simulink model "PTMotorCU"  (Simulink 7.5)
settings: Solver=ode45  StartTime=0.0  StopTime=inf  RelTol=1e-3
PreLoadFcn:
  | xData = [0 13.5 21 35 50 100];
  | yData = [150 150 95 57 39 20];
InitFcn:
  | xData = [0 0.128];
  | yData = [150 150];
libraries: simulink x7, CarMaker4SL x1
(part 1 of 2)
settings Model: Creator=fh  LastModifiedBy=ml  ExtModeAutoUpdateStatusClock=off
settings DataIOCC: SignalLoggingName=sigsOut
settings OptimizationCC: BooleanDataType=off  InitFltsAndDblsToZero=on
settings DebuggingCC: SaveWithParameterizedLinksMsg=none  SignalResolutionControl=TryResolveAllWithWarning  SolverPrmCheckMsg=none  MultiTaskDSMMsg=warning  MultiTaskCondExecSysMsg=none
settings HardwareCC: TargetUnknown=on
settings RTWCC: IncludeERTFirstTime=on
settings CodeAppCC: MaxIdLength=63
settings GRTTargetCC: TargetFcnLib=ansi_tfl_tmw.mat

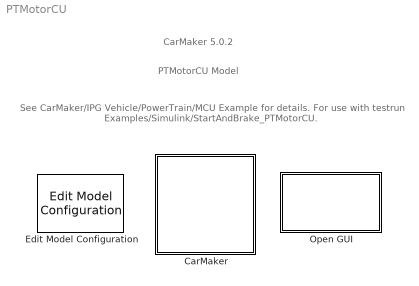
== system PTMotorCU ==
  note: PTMotorCU Model
  note: See CarMaker/IPG Vehicle/PowerTrain/MCU Example for details.
      | For use with testrun Examples/Simulink/StartAndBrake_PTMotorCU.
  note: CarMaker 5.0.2
  CarMaker : Subsystem  TreatAsAtomicUnit=on
      mask Display: image(imread('CarMaker4SLss.bmp'));
  Edit Model Configuration : CarMaker4SL/Edit Model Configuration
  Open GUI : Subsystem  LoadFcn=if ~length(which('cmcmd')), cmenv; end
      settings: OpenFcn=cmblockmagic('gui_fix_display'); CM_Simulink
      mask Display: image(imread('CarMakerGUI.bmp'));

== system PTMotorCU/CarMaker ==
  CM_FIRST : Subsystem
  CM_LAST : Subsystem
  DrivMan : Subsystem
  Ground : Ground
  IPG Vehicle : Subsystem  TreatAsAtomicUnit=on
  Terminator : Terminator
  VehicleControl : Subsystem
  wires:
  DrivMan/2(DrivMan.Out) -> VehicleControl/2(DrivMan.In)
  DrivMan/1(Sync_Out) -> VehicleControl/1(Sync_In)
  CM_FIRST/2(Env.Misc) -> DrivMan/2(Env.Misc)
  CM_FIRST/1(Sync_Out) -> DrivMan/1(Sync_In)
  CM_LAST/1(Sync_Out) -> Terminator/1
  Ground/1 -> CM_FIRST/1(Sync_In)
  IPG Vehicle/1(Sync_Out) -> CM_LAST/1(Sync_In)
  VehicleControl/1(Sync_Out) -> IPG Vehicle/1(Sync_In)
  VehicleControl/3(VhclCtrl.Steering) -> IPG Vehicle/3(VhclCtrl.Steering)
  VehicleControl/4(Vhcl.Wheel.In) -> IPG Vehicle/4(Vhcl.Wheel.In)
  VehicleControl/5(Vhcl.Misc) -> IPG Vehicle/5(Vhcl.Misc)
  VehicleControl/6(VhclCtrl.Brake) -> IPG Vehicle/6(VhclCtrl.Brake)
  VehicleControl/7(VhclCtrl.PT) -> IPG Vehicle/7(VhclCtrl.PT)
  VehicleControl/2(Vhcl.Model.Source) -> IPG Vehicle/2(Vhcl.Model.Source)

== system PTMotorCU/Open GUI ==
  S-Function : S-Function  FunctionName=cm_gui  EnableBusSupport=off

== system PTMotorCU/CarMaker/CM_FIRST ==
  Sync_In : Inport  OutDataType=sfix(16)  OutScaling=2^0
  Bus Creator1 : BusCreator  Inputs=9
  Demux : Demux  Outputs=9
  Environment : S-Function  FunctionName=CM_Sfun  Parameters='Environment'  EnableBusSupport=off
  IoIn : S-Function  FunctionName=CM_Sfun  Parameters='IoIn'  EnableBusSupport=off
  Sync_Out : Outport  OutDataType=sfix(16)  OutScaling=2^0
  Env.Misc : Outport  Port=2  OutDataType=sfix(16)  OutScaling=2^0
  wires:
  Demux/9 -> Bus Creator1/9  "Env WindVel_tot z"
  Demux/8 -> Bus Creator1/8  "Env WindVel_tot y"
  Demux/7 -> Bus Creator1/7  "Env WindVel_tot x"
  Demux/6 -> Bus Creator1/6  "Env SolarRadiation"
  Demux/5 -> Bus Creator1/5  "Env Time"
  Sync_In/1 -> IoIn/1
  IoIn/1 -> Environment/1
  Environment/1 -> Sync_Out/1
  Demux/1 -> Bus Creator1/1  "Env Temperature"
  Demux/2 -> Bus Creator1/2  "Env AirDensity"
  Demux/3 -> Bus Creator1/3  "Env AirPressure"
  Demux/4 -> Bus Creator1/4  "Env AirHumidity"
  Environment/2 -> Demux/1
  Bus Creator1/1 -> Env.Misc/1

== system PTMotorCU/CarMaker/CM_LAST ==
  Sync_In : Inport  OutDataType=sfix(16)  OutScaling=2^0
  CM_User : S-Function  FunctionName=CM_Sfun  Parameters='CM_User'  EnableBusSupport=off
  IoOut : S-Function  FunctionName=CM_Sfun  Parameters='IoOut'  EnableBusSupport=off
  Sync_Out : Outport  OutDataType=sfix(16)  OutScaling=2^0
  wires:
  IoOut/1 -> Sync_Out/1
  CM_User/1 -> IoOut/1
  Sync_In/1 -> CM_User/1

== system PTMotorCU/CarMaker/DrivMan ==
  note: There's rarely a reason to override DrivMan signals.
      | Use the VehicleControl interface for this purpose.
  Sync_In : Inport  OutDataType=sfix(16)  OutScaling=2^0
  Env.Misc : Inport  Port=2  OutDataType=sfix(16)  OutScaling=2^0
  BusCreator : BusCreator  Inputs=17
  Demux : Demux  Outputs=17
  DrivMan : S-Function  FunctionName=CM_Sfun  Parameters='DrivMan'  EnableBusSupport=off
  Sync_Out : Outport  OutDataType=sfix(16)  OutScaling=2^0
  DrivMan.Out : Outport  Port=2  OutDataType=sfix(16)  OutScaling=2^0
  wires:
  DrivMan/2 -> Demux/1
  BusCreator/1 -> DrivMan.Out/1
  DrivMan/1 -> Sync_Out/1
  Sync_In/1 -> DrivMan/1
  Env.Misc/1 -> DrivMan/2
  Demux/1 -> BusCreator/1  "DrivMan SST"
  Demux/2 -> BusCreator/2  "DrivMan Key"
  Demux/3 -> BusCreator/3  "DrivMan UserSignal0"
  Demux/4 -> BusCreator/4  "DrivMan UserSignal1"
  Demux/5 -> BusCreator/5  "DrivMan UserSignal2"
  Demux/6 -> BusCreator/6  "DrivMan UserSignal3"
  Demux/7 -> BusCreator/7  "DrivMan UserSignal4"
  Demux/8 -> BusCreator/8  "DrivMan SelectorCtrl"
  Demux/9 -> BusCreator/9  "DrivMan GearNo"
  Demux/10 -> BusCreator/10  "DrivMan Brake"
  Demux/11 -> BusCreator/11  "DrivMan BrakePark"
  Demux/12 -> BusCreator/12  "DrivMan Clutch"
  Demux/13 -> BusCreator/13  "DrivMan Gas"
  Demux/14 -> BusCreator/14  "DrivMan Steering Ang"
  Demux/15 -> BusCreator/15  "DrivMan Steering AngVel"
  Demux/16 -> BusCreator/16  "DrivMan Steering AngAcc"
  Demux/17 -> BusCreator/17  "DrivMan Steering Trq"

== system PTMotorCU/CarMaker/IPG Vehicle ==
  Sync_In : Inport  OutDataType=sfix(16)  OutScaling=2^0
  Vhcl.Model.Source : Inport  Port=2  OutDataType=sfix(16)  OutScaling=2^0
  VhclCtrl.Steering : Inport  Port=3  OutDataType=sfix(16)  OutScaling=2^0
  Vhcl.Wheel.In : Inport  Port=4  OutDataType=sfix(16)  OutScaling=2^0
  Vhcl.Misc : Inport  Port=5  OutDataType=sfix(16)  OutScaling=2^0
  VhclCtrl.Brake : Inport  Port=6  OutDataType=sfix(16)  OutScaling=2^0
  VhclCtrl.PT : Inport  Port=7  OutDataType=sfix(16)  OutScaling=2^0
  Brake : Subsystem
  CarAndTrailer : Subsystem
  PowerTrain : Subsystem
  Stop Simulation : Stop
  VehicleSource_BuiltIn : simulink/Logic and Bit Operations/Compare To Constant  SystemSampleTime=-1  relop=~=  const=1  LogicOutDataTypeMode=boolean  ZeroCross=off
  Sync_Out : Outport  OutDataType=sfix(16)  OutScaling=2^0
  wires:
  VhclCtrl.PT/1 -> PowerTrain/3(VhclCtrl.PT)
  CarAndTrailer/1(Sync_Out) -> Brake/1(Sync_In)
  CarAndTrailer/2(Brake.IF.In) -> Brake/2(Brake.IF.In)
  VhclCtrl.Brake/1 -> Brake/3(VhclCtrl.Brake)
  PowerTrain/1(Sync_Out) -> Sync_Out/1
  Vhcl.Misc/1 -> CarAndTrailer/4(Vhcl.Misc)
  Vhcl.Wheel.In/1 -> CarAndTrailer/3(Vhcl.Wheel.In)
  VhclCtrl.Steering/1 -> CarAndTrailer/2(VhclCtrl.Steering)
  Sync_In/1 -> CarAndTrailer/1(Sync_In)
  Vhcl.Model.Source/1 -> VehicleSource_BuiltIn/1
  VehicleSource_BuiltIn/1 -> Stop Simulation/1
  Brake/1(Sync_Out) -> PowerTrain/1(Sync_In)
  Brake/2(Vhcl.Wheel.PT) -> PowerTrain/2(Vhcl.Wheel.PT)

== system PTMotorCU/CarMaker/VehicleControl ==
  note: <Your model here>
  note: When implementing a vehicle control model,
      | be sure to add '-disablevehiclecontrol' to the command line arguments
      | in the CarMaker Model Configuration block.
      | Otherwise your model will possibly not see the original DrivMan signals
      | on its inputs, but those of a currently activated C-coded vehicle control model instead.
  Sync_In : Inport  OutDataType=sfix(16)  OutScaling=2^0
  DrivMan.In : Inport  Port=2  OutDataType=sfix(16)  OutScaling=2^0
  Bus Creator2 : BusCreator  Inputs=2
  CreateBus Vhcl.Misc : Subsystem
  CreateBus Vhcl.Wheel.In : Subsystem
  CreateBus VhclCtrl : Subsystem
  CreateBus VhclCtrl.PT : Subsystem
  CreateBus VhclCtrl.Steering : Subsystem
  Demux2 : Demux  Outputs=2
  VehicleControl : S-Function  FunctionName=CM_Sfun  Parameters='VehicleControl'  EnableBusSupport=off
  VehicleControlUpd : S-Function  FunctionName=CM_Sfun  Parameters='VehicleControlUpd'  EnableBusSupport=off
  Sync_Out : Outport  OutDataType=sfix(16)  OutScaling=2^0
  Vhcl.Model.Source : Outport  Port=2  OutDataType=sfix(16)  OutScaling=2^0
  VhclCtrl.Steering : Outport  Port=3  OutDataType=sfix(16)  OutScaling=2^0
  Vhcl.Wheel.In : Outport  Port=4  OutDataType=sfix(16)  OutScaling=2^0
  Vhcl.Misc : Outport  Port=5  OutDataType=sfix(16)  OutScaling=2^0
  VhclCtrl.Brake : Outport  Port=6  OutDataType=sfix(16)  OutScaling=2^0
  VhclCtrl.PT : Outport  Port=7  OutDataType=sfix(16)  OutScaling=2^0
  wires:
  CreateBus VhclCtrl/1(Out) -> VehicleControlUpd/2
  VehicleControl/2 -> CreateBus VhclCtrl/1(In)
  VehicleControlUpd/2 -> Vhcl.Model.Source/1
  VehicleControlUpd/4 -> CreateBus Vhcl.Wheel.In/1(In1)
  VehicleControlUpd/5 -> CreateBus Vhcl.Misc/1(In1)
  VehicleControlUpd/6 -> Demux2/1
  VehicleControlUpd/7 -> CreateBus VhclCtrl.PT/1(In1)
  VehicleControlUpd/3 -> CreateBus VhclCtrl.Steering/1(In1)
  CreateBus Vhcl.Misc/1(Out1) -> Vhcl.Misc/1
  CreateBus Vhcl.Wheel.In/1(Out1) -> Vhcl.Wheel.In/1
  DrivMan.In/1 -> VehicleControl/2
  VehicleControl/1 -> VehicleControlUpd/1
  Sync_In/1 -> VehicleControl/1
  CreateBus VhclCtrl.PT/1(Out1) -> VhclCtrl.PT/1
  Bus Creator2/1 -> VhclCtrl.Brake/1
  CreateBus VhclCtrl.Steering/1(Out1) -> VhclCtrl.Steering/1
  VehicleControlUpd/1 -> Sync_Out/1
  Demux2/2 -> Bus Creator2/2  "VhclCtrl BrakePark"
  Demux2/1 -> Bus Creator2/1  "VhclCtrl Brake"

== system PTMotorCU/CarMaker/IPG Vehicle/Brake ==
  note: When replacing the entire braking system,
      | be sure to add '-disablebrake' to the command line arguments
      | in the CarMaker Model Configuration block.
  note: <Your model here>
  Sync_In : Inport  OutDataType=sfix(16)  OutScaling=2^0
  Brake.IF.In : Inport  Port=2  OutDataType=sfix(16)  OutScaling=2^0
  VhclCtrl.Brake : Inport  Port=3  OutDataType=sfix(16)  OutScaling=2^0
  Brake : S-Function  FunctionName=CM_Sfun  Parameters='Brake'  EnableBusSupport=off
  BrakeUpd : S-Function  FunctionName=CM_Sfun  Parameters='BrakeUpd'  EnableBusSupport=off
  BusCreator : BusCreator  Inputs=12
  CreateBus Vhcl.Wheel.PT : Subsystem
  Demux : Demux  Outputs=12
  Sync_Out : Outport  OutDataType=sfix(16)  OutScaling=2^0
  Vhcl.Wheel.PT : Outport  Port=2  OutDataType=sfix(16)  OutScaling=2^0
  wires:
  CreateBus Vhcl.Wheel.PT/1(Out) -> Vhcl.Wheel.PT/1
  BrakeUpd/2 -> CreateBus Vhcl.Wheel.PT/1(In)
  Demux/1 -> BusCreator/1  "Brake IF Trq_WB FL"
  Demux/2 -> BusCreator/2  "Brake IF Trq_WB FR"
  Demux/3 -> BusCreator/3  "Brake IF Trq_WB RL"
  Demux/4 -> BusCreator/4  "Brake IF Trq_WB RR"
  Demux/5 -> BusCreator/5  "Brake IF Trq_PB FL"
  Demux/6 -> BusCreator/6  "Brake IF Trq_PB FR"
  Demux/7 -> BusCreator/7  "Brake IF Trq_PB RL"
  Demux/8 -> BusCreator/8  "Brake IF Trq_PB RR"
  Demux/9 -> BusCreator/9  "Brake IF Trq_Reg_trg FL"
  Demux/10 -> BusCreator/10  "Brake IF Trq_Reg_trg FR"
  Demux/11 -> BusCreator/11  "Brake IF Trq_Reg_trg RL"
  Demux/12 -> BusCreator/12  "Brake IF Trq_Reg_trg RR"
  Sync_In/1 -> Brake/1
  BusCreator/1 -> BrakeUpd/2
  Brake/2 -> Demux/1
  VhclCtrl.Brake/1 -> Brake/3
  Brake.IF.In/1 -> Brake/2
  Brake/1 -> BrakeUpd/1  "Sync"
  BrakeUpd/1 -> Sync_Out/1

== system PTMotorCU/CarMaker/IPG Vehicle/CarAndTrailer ==
  Sync_In : Inport  OutDataType=sfix(16)  OutScaling=2^0
  VhclCtrl.Steering : Inport  Port=2  OutDataType=sfix(16)  OutScaling=2^0
  Vhcl.Wheel.In : Inport  Port=3  OutDataType=sfix(16)  OutScaling=2^0
  Vhcl.Misc : Inport  Port=4  OutDataType=sfix(16)  OutScaling=2^0
  CarAndTrailerUpd : Subsystem
  Forces : Subsystem
  Ground : Ground
  Kinematics : Subsystem
  Kinetics : Subsystem
  Steering : Subsystem
  Terminator : Terminator
  Terminator1 : Terminator
  Trailer : Subsystem
  Sync_Out : Outport  OutDataType=sfix(16)  OutScaling=2^0
  Brake.IF.In : Outport  Port=2  OutDataType=sfix(16)  OutScaling=2^0
  wires:
  Kinematics/9(lBuf) -> Forces/9(lBuf)
  Forces/12(FBuf) -> Kinetics/12(FBuf)
  Kinematics/8(lStabi) -> Forces/8(lStabi)
  Kinematics/1(Sync_Out) -> Forces/1(Sync_In)
  Kinematics/2(TireFL_In) -> Forces/2(TireFL_In)
  Kinematics/3(TireFR_In) -> Forces/3(TireFR_In)
  Kinematics/4(TireRL_In) -> Forces/4(TireRL_In)
  Kinematics/5(TireRR_In) -> Forces/5(TireRR_In)
  Forces/1(Sync_Out) -> Kinetics/1(Sync_In)
  Forces/3(Car.Aero) -> Kinetics/3(Car.Aero)
  Kinematics/7(vDamp) -> Forces/7(vDamp)
  Kinematics/6(lSpring) -> Forces/6(lSpring)
  Forces/2(Car.Virtual) -> Kinetics/2(Car.Virtual)
  Forces/4(Car.Load) -> Kinetics/4(Car.Load)
  Forces/5(TireFL_Out) -> Kinetics/5(TireFL.Out)
  Forces/6(TireFR_Out) -> Kinetics/6(TireFR.Out)
  Forces/7(TireRL_Out) -> Kinetics/7(TireRL.Out)
  Forces/8(TireRR_Out) -> Kinetics/8(TireRR.Out)
  Forces/9(FSpring) -> Kinetics/9(FSpring)
  Forces/10(FDamp) -> Kinetics/10(FDamp)
  Forces/11(FStabi) -> Kinetics/11(FStabi)
  Ground/1 -> CarAndTrailerUpd/10(Vhcl.Fr1A)
  Kinetics/1(Sync_Out) -> Trailer/1(Sync_In)
  Steering/1(Sync_Out) -> Kinematics/1(Sync_In)
  Sync_In/1 -> Steering/1(Sync_In)
  VhclCtrl.Steering/1 -> Steering/2(VhclCtrl.Steering)
  Kinetics/2(Trailer.Load) -> Trailer/2(Trailer.Load)
  Kinetics/3(Car.Hitch) -> Trailer/3(Car.Hitch)
  Kinetics/4(Car.Fr1) -> Trailer/4(Car.Fr1)
  Steering/2(Steer.IF) -> Kinematics/2(Steer.IF)
  Kinetics/5(Car.Trq_T2W) -> Trailer/5(Car.Trq_T2W)
  Kinetics/6(WheelCarrier.Misc) -> Trailer/6(WheelCarrier.Misc)
  Vhcl.Wheel.In/1 -> Terminator/1
  Vhcl.Misc/1 -> Terminator1/1
  CarAndTrailerUpd/1(Sync_Out) -> Sync_Out/1
  CarAndTrailerUpd/2(Brake.IF.In) -> Brake.IF.In/1
  Trailer/1(Sync_Out) -> CarAndTrailerUpd/1(Sync_In)
  Trailer/2(Vhcl.Steering) -> CarAndTrailerUpd/2(Vhcl.Steering)
  Trailer/3(Vhcl.Motion) -> CarAndTrailerUpd/3(Vhcl.Motion)
  Trailer/4(Vhcl.PoI) -> CarAndTrailerUpd/4(Vhcl.PoI)
  Trailer/5(Vhcl.Wheel.FL) -> CarAndTrailerUpd/5(Vhcl.Wheel.FL)
  Trailer/6(Vhcl.Wheel.FR) -> CarAndTrailerUpd/6(Vhcl.Wheel.FR)
  Trailer/7(Vhcl.Wheel.RL) -> CarAndTrailerUpd/7(Vhcl.Wheel.RL)
  Trailer/8(Vhcl.Wheel.RR) -> CarAndTrailerUpd/8(Vhcl.Wheel.RR)
  Trailer/9(Car.Hitch.FrcTrq) -> CarAndTrailerUpd/9(Car.Hitch.FrcTrq)

== system PTMotorCU/CarMaker/IPG Vehicle/PowerTrain ==
  note: <Your model here>
  note: When replacing the entire powertrain,
      | be sure to add '-disablepowertrain' to the command line arguments
      | in the CarMaker Model Configuration block.
  Sync_In : Inport  OutDataType=sfix(16)  OutScaling=2^0
  Vhcl.Wheel.PT : Inport  Port=2  OutDataType=sfix(16)  OutScaling=2^0
  VhclCtrl.PT : Inport  Port=3  OutDataType=sfix(16)  OutScaling=2^0
  BusCreator : BusCreator  Inputs=40
  Demux : Demux  Outputs=40
  MCU Example : Subsystem
  PowerTrain : S-Function  FunctionName=CM_Sfun  Parameters='PowerTrain'  EnableBusSupport=off
  PowerTrainUpd : S-Function  FunctionName=CM_Sfun  Parameters='PowerTrainUpd'  EnableBusSupport=off
  Sync_Out : Outport  OutDataType=sfix(16)  OutScaling=2^0
  wires:
  Vhcl.Wheel.PT/1 -> PowerTrain/2
  VhclCtrl.PT/1 -> PowerTrain/3
  Demux/40 -> BusCreator/40  "PT IF WRR Trq_BrakeReg_max"
  Demux/39 -> BusCreator/39  "PT IF WRR Trq_BrakeReg"
  Demux/38 -> BusCreator/38  "PT IF WRR Trq_Supp2WC"
  Demux/37 -> BusCreator/37  "PT IF WRR Trq_Drive"
  Demux/36 -> BusCreator/36  "PT IF WRR Trq_B2W"
  Demux/35 -> BusCreator/35  "PT IF WRR rotv"
  Demux/34 -> BusCreator/34  "PT IF WRR rot"
  Demux/33 -> BusCreator/33  "PT IF WRL Trq_BrakeReg_max"
  Demux/32 -> BusCreator/32  "PT IF WRL Trq_BrakeReg"
  Demux/31 -> BusCreator/31  "PT IF WRL Trq_Supp2WC"
  Demux/30 -> BusCreator/30  "PT IF WRL Trq_Drive"
  Demux/29 -> BusCreator/29  "PT IF WRL Trq_B2W"
  Demux/28 -> BusCreator/28  "PT IF WRL rotv"
  Demux/27 -> BusCreator/27  "PT IF WRL rot"
  Demux/26 -> BusCreator/26  "PT IF WFR Trq_BrakeReg_max"
  Demux/25 -> BusCreator/25  "PT IF WFR Trq_BrakeReg"
  Demux/24 -> BusCreator/24  "PT IF WFR Trq_Supp2WC"
  Demux/23 -> BusCreator/23  "PT IF WFR Trq_Drive"
  Demux/22 -> BusCreator/22  "PT IF WFR Trq_B2W"
  Demux/21 -> BusCreator/21  "PT IF WFR rotv"
  Demux/20 -> BusCreator/20  "PT IF WFR rot"
  Demux/19 -> BusCreator/19  "PT IF WFL Trq_BrakeReg_max"
  Demux/18 -> BusCreator/18  "PT IF WFL Trq_BrakeReg"
  Demux/17 -> BusCreator/17  "PT IF WFL Trq_Supp2WC"
  Demux/16 -> BusCreator/16  "PT IF WFL Trq_Drive"
  Demux/15 -> BusCreator/15  "PT IF WFL Trq_B2W"
  Demux/14 -> BusCreator/14  "PT IF WFL rotv"
  Demux/13 -> BusCreator/13  "PT IF WFL rot"
  Demux/12 -> BusCreator/12  "PT IF DL_iDiff_mean"
  Demux/11 -> BusCreator/11  "PT IF Trq_Supp2BdyEng y"
  Demux/10 -> BusCreator/10  "PT IF Trq_Supp2BdyEng x"
  Demux/9 -> BusCreator/9  "PT IF Trq_Supp2Bdy1 z"
  Demux/8 -> BusCreator/8  "PT IF Trq_Supp2Bdy1 y"
  Demux/7 -> BusCreator/7  "PT IF Trq_Supp2Bdy1 x"
  Demux/6 -> BusCreator/6  "PT IF Engine_Trq (EngineControl)"
  Demux/5 -> BusCreator/5  "PT IF Engine_rotv"
  Demux/4 -> BusCreator/4  "PT IF GearNo"
  Demux/3 -> BusCreator/3  "PT IF OperationError"
  Demux/2 -> BusCreator/2  "PT IF OperationState"
  Demux/1 -> BusCreator/1  "PT IF Ignition"
  BusCreator/1 -> PowerTrainUpd/2
  PowerTrain/1 -> PowerTrainUpd/1, MCU Example/1(Sync_In)  "Sync"
  PowerTrainUpd/1 -> Sync_Out/1
  PowerTrain/2 -> Demux/1
  Sync_In/1 -> PowerTrain/1

== system PTMotorCU/CarMaker/VehicleControl/CreateBus Vhcl.Misc ==
  In1 : Inport  OutDataType=sfix(16)  OutScaling=2^0
  Bus Creator5 : BusCreator  Inputs=11
  Demux5 : Demux  Outputs=11
  Out1 : Outport  OutDataType=sfix(16)  OutScaling=2^0
  wires:
  Demux5/11 -> Bus Creator5/11  "Vhcl Wind_vel_0 z"
  Demux5/10 -> Bus Creator5/10  "Vhcl Wind_vel_0 y"
  Demux5/9 -> Bus Creator5/9  "Vhcl Wind_vel_0 x"
  Demux5/8 -> Bus Creator5/8  "Vhcl DL2BdyEng y"
  Demux5/7 -> Bus Creator5/7  "Vhcl DL2BdyEng x"
  Demux5/6 -> Bus Creator5/6  "Vhcl TrqDL2Bdy1B z"
  Demux5/5 -> Bus Creator5/5  "Vhcl TrqDL2Bdy1B y"
  Demux5/4 -> Bus Creator5/4  "Vhcl TrqDL2Bdy1B x"
  Demux5/3 -> Bus Creator5/3  "Vhcl Trq_DL2Bdy1 z"
  In1/1 -> Demux5/1
  Bus Creator5/1 -> Out1/1
  Demux5/2 -> Bus Creator5/2  "Vhcl Trq_DL2Bdy1 y"
  Demux5/1 -> Bus Creator5/1  "Vhcl Trq_DL2Bdy1 x"

== system PTMotorCU/CarMaker/VehicleControl/CreateBus Vhcl.Wheel.In ==
  In1 : Inport  OutDataType=sfix(16)  OutScaling=2^0
  Bus Creator1 : BusCreator  Inputs=12
  Demux1 : Demux  Outputs=12
  Out1 : Outport  OutDataType=sfix(16)  OutScaling=2^0
  wires:
  Demux1/12 -> Bus Creator1/12  "Vhcl Wheel RR rotv"
  Demux1/11 -> Bus Creator1/11  "Vhcl Wheel RR Trq_DL2WC"
  Demux1/10 -> Bus Creator1/10  "Vhcl Wheel RR Trq_B2WC"
  Demux1/9 -> Bus Creator1/9  "Vhcl Wheel RL rotv"
  Demux1/8 -> Bus Creator1/8  "Vhcl Wheel RL Trq_DL2WC"
  Demux1/7 -> Bus Creator1/7  "Vhcl Wheel RL Trq_B2WC"
  Demux1/6 -> Bus Creator1/6  "Vhcl Wheel FR rotv"
  Demux1/5 -> Bus Creator1/5  "Vhcl Wheel FR Trq_DL2WC"
  Demux1/4 -> Bus Creator1/4  "Vhcl Wheel FR Trq_B2WC"
  Demux1/3 -> Bus Creator1/3  "Vhcl Wheel FL rotv"
  In1/1 -> Demux1/1
  Bus Creator1/1 -> Out1/1
  Demux1/2 -> Bus Creator1/2  "Vhcl Wheel FL Trq_DL2WC"
  Demux1/1 -> Bus Creator1/1  "Vhcl Wheel FL Trq_B2WC"

== system PTMotorCU/CarMaker/VehicleControl/CreateBus VhclCtrl ==
  In : Inport
  BusCreator : BusCreator  Inputs=29
  Demux : Demux  Outputs=29
  Out : Outport
  wires:
  In/1 -> Demux/1
  BusCreator/1 -> Out/1
  Demux/1 -> BusCreator/1  "VhclCtrl SST"
  Demux/2 -> BusCreator/2  "VhclCtrl Key"
  Demux/3 -> BusCreator/3  "VhclCtrl UserSignal0"
  Demux/4 -> BusCreator/4  "VhclCtrl UserSignal1"
  Demux/5 -> BusCreator/5  "VhclCtrl UserSignal2"
  Demux/6 -> BusCreator/6  "VhclCtrl UserSignal3"
  Demux/7 -> BusCreator/7  "VhclCtrl UserSignal4"
  Demux/8 -> BusCreator/8  "VhclCtrl GearNo"
  Demux/9 -> BusCreator/9  "VhclCtrl SelectorCtrl"
  Demux/10 -> BusCreator/10  "VhclCtrl Brake"
  Demux/11 -> BusCreator/11  "VhclCtrl BrakePark"
  Demux/12 -> BusCreator/12  "VhclCtrl Clutch"
  Demux/13 -> BusCreator/13  "VhclCtrl Gas"
  Demux/14 -> BusCreator/14  "VhclCtrl Steering Ang"
  Demux/15 -> BusCreator/15  "VhclCtrl Steering AngVel"
  Demux/16 -> BusCreator/16  "VhclCtrl Steering AngAcc"
  Demux/17 -> BusCreator/17  "VhclCtrl Steering Trq"
  Demux/18 -> BusCreator/18  "VhclCtrl Lights LowBeam"
  Demux/19 -> BusCreator/19  "VhclCtrl Lights HighBeam"
  Demux/20 -> BusCreator/20  "VhclCtrl Lights Daytime"
  Demux/21 -> BusCreator/21  "VhclCtrl Lights ParkL"
  Demux/22 -> BusCreator/22  "VhclCtrl Lights ParkR"
  Demux/23 -> BusCreator/23  "VhclCtrl Lights IndL"
  Demux/24 -> BusCreator/24  "VhclCtrl Lights IndR"
  Demux/25 -> BusCreator/25  "VhclCtrl Lights FogFrontL"
  Demux/26 -> BusCreator/26  "VhclCtrl Lights FogFrontR"
  Demux/27 -> BusCreator/27  "VhclCtrl Lights FogRear"
  Demux/28 -> BusCreator/28  "VhclCtrl Lights Brake"
  Demux/29 -> BusCreator/29  "VhclCtrl Lights Reverse"

== system PTMotorCU/CarMaker/VehicleControl/CreateBus VhclCtrl.PT ==
  In1 : Inport
  BusCreator : BusCreator  Inputs=11
  Demux : Demux  Outputs=11
  Out1 : Outport
  wires:
  In1/1 -> Demux/1
  BusCreator/1 -> Out1/1
  Demux/1 -> BusCreator/1  "VhclCtrl SST"
  Demux/2 -> BusCreator/2  "VhclCtrl Key"
  Demux/3 -> BusCreator/3  "VhclCtrl UserSignal0"
  Demux/4 -> BusCreator/4  "VhclCtrl UserSignal1"
  Demux/5 -> BusCreator/5  "VhclCtrl UserSignal2"
  Demux/6 -> BusCreator/6  "VhclCtrl UserSignal3"
  Demux/7 -> BusCreator/7  "VhclCtrl UserSignal4"
  Demux/8 -> BusCreator/8  "VhclCtrl GearNo"
  Demux/9 -> BusCreator/9  "VhclCtrl SelectorCtrl"
  Demux/10 -> BusCreator/10  "VhclCtrl Clutch"
  Demux/11 -> BusCreator/11  "VhclCtrl Gas"

== system PTMotorCU/CarMaker/VehicleControl/CreateBus VhclCtrl.Steering ==
  In1 : Inport  OutDataType=sfix(16)  OutScaling=2^0
  Bus Creator : BusCreator  Inputs=5
  Demux : Demux  Outputs=5
  Out1 : Outport  OutDataType=sfix(16)  OutScaling=2^0
  wires:
  In1/1 -> Demux/1
  Bus Creator/1 -> Out1/1
  Demux/1 -> Bus Creator/1  "VhclCtrl Steering Ang"
  Demux/5 -> Bus Creator/5  "VhclCtrl Steering ByTrq"
  Demux/3 -> Bus Creator/3  "VhclCtrl Steering AngAcc"
  Demux/2 -> Bus Creator/2  "VhclCtrl Steering AngVel"
  Demux/4 -> Bus Creator/4  "VhclCtrl Steering Trq"

== system PTMotorCU/CarMaker/IPG Vehicle/Brake/CreateBus Vhcl.Wheel.PT ==
  In : Inport
  BusCreator : BusCreator  Inputs=16
  Demux : Demux  Outputs=16
  Out : Outport
  wires:
  In/1 -> Demux/1
  BusCreator/1 -> Out/1
  Demux/1 -> BusCreator/1  "Vhcl Wheel FL Trq_Brake"
  Demux/2 -> BusCreator/2  "Vhcl Wheel FL Trq_BrakeReg_trg"
  Demux/3 -> BusCreator/3  "Vhcl Wheel FL Trq_T2W"
  Demux/4 -> BusCreator/4  "Vhcl Wheel FL WhlBearing"
  Demux/5 -> BusCreator/5  "Vhcl Wheel FR Trq_Brake"
  Demux/6 -> BusCreator/6  "Vhcl Wheel FR Trq_BrakeReg_trg"
  Demux/7 -> BusCreator/7  "Vhcl Wheel FR Trq_T2W"
  Demux/8 -> BusCreator/8  "Vhcl Wheel FR WhlBearing"
  Demux/9 -> BusCreator/9  "Vhcl Wheel RL Trq_Brake"
  Demux/10 -> BusCreator/10  "Vhcl Wheel RL Trq_BrakeReg_trg"
  Demux/11 -> BusCreator/11  "Vhcl Wheel RL Trq_T2W"
  Demux/12 -> BusCreator/12  "Vhcl Wheel RL WhlBearing"
  Demux/13 -> BusCreator/13  "Vhcl Wheel RR Trq_Brake"
  Demux/14 -> BusCreator/14  "Vhcl Wheel RR Trq_BrakeReg_trg"
  Demux/15 -> BusCreator/15  "Vhcl Wheel RR Trq_T2W"
  Demux/16 -> BusCreator/16  "Vhcl Wheel RR WhlBearing"

== system PTMotorCU/CarMaker/IPG Vehicle/CarAndTrailer/CarAndTrailerUpd ==
  Sync_In : Inport  OutDataType=sfix(16)  OutScaling=2^0
  Vhcl.Steering : Inport  Port=2  OutDataType=sfix(16)  OutScaling=2^0
  Vhcl.Motion : Inport  Port=3  OutDataType=sfix(16)  OutScaling=2^0
  Vhcl.PoI : Inport  Port=4  OutDataType=sfix(16)  OutScaling=2^0
  Vhcl.Wheel.FL : Inport  Port=5  OutDataType=sfix(16)  OutScaling=2^0
  Vhcl.Wheel.FR : Inport  Port=6  OutDataType=sfix(16)  OutScaling=2^0
  Vhcl.Wheel.RL : Inport  Port=7  OutDataType=sfix(16)  OutScaling=2^0
  Vhcl.Wheel.RR : Inport  Port=8  OutDataType=sfix(16)  OutScaling=2^0
  Car.Hitch.FrcTrq : Inport  Port=9  OutDataType=sfix(16)  OutScaling=2^0
  Vhcl.Fr1A : Inport  Port=10  OutDataType=sfix(16)  OutScaling=2^0
  CarAndTrailerUpd : S-Function  FunctionName=CM_Sfun  Parameters='CarAndTrUpd'  EnableBusSupport=off
  CreateBus Brake.IF.In : Subsystem
  Sync_Out : Outport  OutDataType=sfix(16)  OutScaling=2^0
  Brake.IF.In : Outport  Port=2  OutDataType=sfix(16)  OutScaling=2^0
  wires:
  Sync_In/1 -> CarAndTrailerUpd/1
  CarAndTrailerUpd/1 -> Sync_Out/1
  CreateBus Brake.IF.In/1(Out) -> Brake.IF.In/1
  CarAndTrailerUpd/2 -> CreateBus Brake.IF.In/1(In)
  Vhcl.Wheel.RL/1 -> CarAndTrailerUpd/7
  Vhcl.Wheel.RR/1 -> CarAndTrailerUpd/8
  Car.Hitch.FrcTrq/1 -> CarAndTrailerUpd/9
  Vhcl.Wheel.FR/1 -> CarAndTrailerUpd/6
  Vhcl.Wheel.FL/1 -> CarAndTrailerUpd/5
  Vhcl.PoI/1 -> CarAndTrailerUpd/4
  Vhcl.Motion/1 -> CarAndTrailerUpd/3
  Vhcl.Steering/1 -> CarAndTrailerUpd/2
  Vhcl.Fr1A/1 -> CarAndTrailerUpd/10  "user vehicle only"

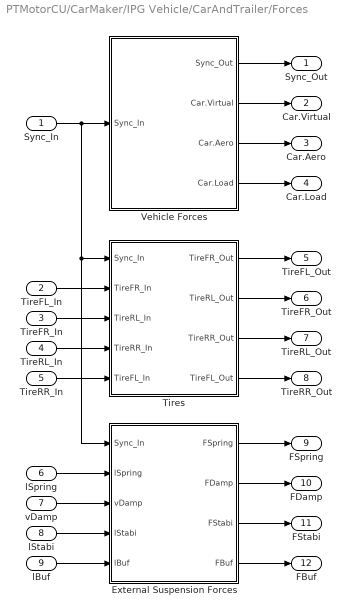
== system PTMotorCU/CarMaker/IPG Vehicle/CarAndTrailer/Forces ==
  Sync_In : Inport  OutDataType=sfix(16)  OutScaling=2^0
  TireFL_In : Inport  Port=2  OutDataType=sfix(16)  OutScaling=2^0
  TireFR_In : Inport  Port=3  OutDataType=sfix(16)  OutScaling=2^0
  TireRL_In : Inport  Port=4  OutDataType=sfix(16)  OutScaling=2^0
  TireRR_In : Inport  Port=5  OutDataType=sfix(16)  OutScaling=2^0
  lSpring : Inport  Port=6  OutDataType=sfix(16)  OutScaling=2^0
  vDamp : Inport  Port=7  OutDataType=sfix(16)  OutScaling=2^0
  lStabi : Inport  Port=8  OutDataType=sfix(16)  OutScaling=2^0
  lBuf : Inport  Port=9  OutDataType=sfix(16)  OutScaling=2^0
  External Suspension Forces : Subsystem
  Tires : Subsystem
  Vehicle Forces : Subsystem
  Sync_Out : Outport  OutDataType=sfix(16)  OutScaling=2^0
  Car.Virtual : Outport  Port=2  OutDataType=sfix(16)  OutScaling=2^0
  Car.Aero : Outport  Port=3  OutDataType=sfix(16)  OutScaling=2^0
  Car.Load : Outport  Port=4  OutDataType=sfix(16)  OutScaling=2^0
  TireFL_Out : Outport  Port=5  OutDataType=sfix(16)  OutScaling=2^0
  TireFR_Out : Outport  Port=6  OutDataType=sfix(16)  OutScaling=2^0
  TireRL_Out : Outport  Port=7  OutDataType=sfix(16)  OutScaling=2^0
  TireRR_Out : Outport  Port=8  OutDataType=sfix(16)  OutScaling=2^0
  FSpring : Outport  Port=9  OutDataType=sfix(16)  OutScaling=2^0
  FDamp : Outport  Port=10  OutDataType=sfix(16)  OutScaling=2^0
  FStabi : Outport  Port=11  OutDataType=sfix(16)  OutScaling=2^0
  FBuf : Outport  Port=12  OutDataType=sfix(16)  OutScaling=2^0
  wires:
  External Suspension Forces/1(FSpring) -> FSpring/1
  External Suspension Forces/3(FStabi) -> FStabi/1
  lStabi/1 -> External Suspension Forces/4(lStabi)
  vDamp/1 -> External Suspension Forces/3(vDamp)
  External Suspension Forces/2(FDamp) -> FDamp/1
  lSpring/1 -> External Suspension Forces/2(lSpring)
  Vehicle Forces/4(Car.Load) -> Car.Load/1
  Vehicle Forces/3(Car.Aero) -> Car.Aero/1
  Vehicle Forces/2(Car.Virtual) -> Car.Virtual/1
  TireFL_In/1 -> Tires/2(TireFR_In)
  Vehicle Forces/1(Sync_Out) -> Sync_Out/1
  Sync_In/1 -> Vehicle Forces/1(Sync_In), Tires/1(Sync_In), External Suspension Forces/1(Sync_In)
  TireFR_In/1 -> Tires/3(TireRL_In)
  TireRL_In/1 -> Tires/4(TireRR_In)
  TireRR_In/1 -> Tires/5(TireFL_In)
  Tires/1(TireFR_Out) -> TireFL_Out/1
  Tires/2(TireRL_Out) -> TireFR_Out/1
  Tires/3(TireRR_Out) -> TireRL_Out/1
  Tires/4(TireFL_Out) -> TireRR_Out/1
  lBuf/1 -> External Suspension Forces/5(lBuf)
  External Suspension Forces/4(FBuf) -> FBuf/1

== system PTMotorCU/CarMaker/IPG Vehicle/CarAndTrailer/Kinematics ==
  Sync_In : Inport  OutDataType=sfix(16)  OutScaling=2^0
  Steer.IF : Inport  Port=2  OutDataType=sfix(16)  OutScaling=2^0
  Kinematics : S-Function  FunctionName=CM_Sfun  Parameters='Kinematics'  EnableBusSupport=off
  Sync_Out : Outport  OutDataType=sfix(16)  OutScaling=2^0
  TireFL_In : Outport  Port=2  OutDataType=sfix(16)  OutScaling=2^0
  TireFR_In : Outport  Port=3  OutDataType=sfix(16)  OutScaling=2^0
  TireRL_In : Outport  Port=4  OutDataType=sfix(16)  OutScaling=2^0
  TireRR_In : Outport  Port=5  OutDataType=sfix(16)  OutScaling=2^0
  lSpring : Outport  Port=6  OutDataType=sfix(16)  OutScaling=2^0
  vDamp : Outport  Port=7  OutDataType=sfix(16)  OutScaling=2^0
  lStabi : Outport  Port=8  OutDataType=sfix(16)  OutScaling=2^0
  lBuf : Outport  Port=9  OutDataType=sfix(16)  OutScaling=2^0
  wires:
  Steer.IF/1 -> Kinematics/2
  Kinematics/1 -> Sync_Out/1
  Sync_In/1 -> Kinematics/1
  Kinematics/7 -> vDamp/1
  Kinematics/6 -> lSpring/1
  Kinematics/5 -> TireRR_In/1
  Kinematics/4 -> TireRL_In/1
  Kinematics/3 -> TireFR_In/1
  Kinematics/2 -> TireFL_In/1
  Kinematics/8 -> lStabi/1
  Kinematics/9 -> lBuf/1

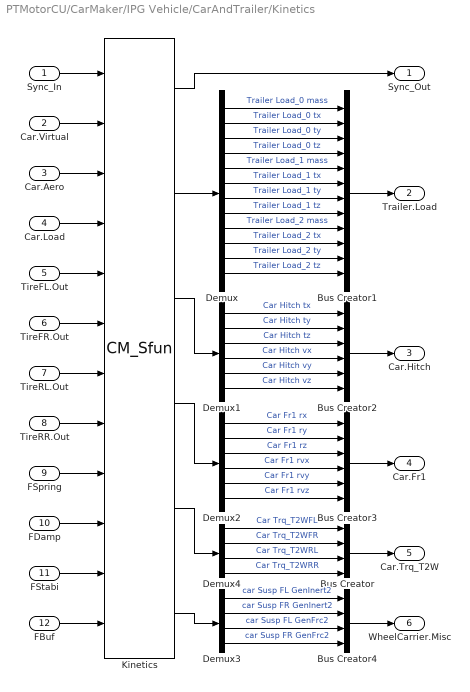
== system PTMotorCU/CarMaker/IPG Vehicle/CarAndTrailer/Kinetics ==
  Sync_In : Inport  OutDataType=sfix(16)  OutScaling=2^0
  Car.Virtual : Inport  Port=2  OutDataType=sfix(16)  OutScaling=2^0
  Car.Aero : Inport  Port=3  OutDataType=sfix(16)  OutScaling=2^0
  Car.Load : Inport  Port=4  OutDataType=sfix(16)  OutScaling=2^0
  TireFL.Out : Inport  Port=5  OutDataType=sfix(16)  OutScaling=2^0
  TireFR.Out : Inport  Port=6  OutDataType=sfix(16)  OutScaling=2^0
  TireRL.Out : Inport  Port=7  OutDataType=sfix(16)  OutScaling=2^0
  TireRR.Out : Inport  Port=8  OutDataType=sfix(16)  OutScaling=2^0
  FSpring : Inport  Port=9  OutDataType=sfix(16)  OutScaling=2^0
  FDamp : Inport  Port=10  OutDataType=sfix(16)  OutScaling=2^0
  FStabi : Inport  Port=11  OutDataType=sfix(16)  OutScaling=2^0
  FBuf : Inport  Port=12  OutDataType=sfix(16)  OutScaling=2^0
  Bus Creator : BusCreator
  Bus Creator1 : BusCreator  Inputs=12
  Bus Creator2 : BusCreator  Inputs=6
  Bus Creator3 : BusCreator  Inputs=6
  Bus Creator4 : BusCreator
  Demux : Demux  Outputs=12
  Demux1 : Demux  Outputs=6
  Demux2 : Demux  Outputs=6
  Demux3 : Demux
  Demux4 : Demux
  Kinetics : S-Function  FunctionName=CM_Sfun  Parameters='Kinetics'  EnableBusSupport=off
  Sync_Out : Outport  OutDataType=sfix(16)  OutScaling=2^0
  Trailer.Load : Outport  Port=2  OutDataType=sfix(16)  OutScaling=2^0
  Car.Hitch : Outport  Port=3  OutDataType=sfix(16)  OutScaling=2^0
  Car.Fr1 : Outport  Port=4  OutDataType=sfix(16)  OutScaling=2^0
  Car.Trq_T2W : Outport  Port=5  OutDataType=sfix(16)  OutScaling=2^0
  WheelCarrier.Misc : Outport  Port=6  OutDataType=sfix(16)  OutScaling=2^0
  wires:
  Kinetics/5 -> Demux4/1
  Kinetics/6 -> Demux3/1
  FStabi/1 -> Kinetics/11
  FDamp/1 -> Kinetics/10
  FSpring/1 -> Kinetics/9
  TireRR.Out/1 -> Kinetics/8
  TireRL.Out/1 -> Kinetics/7
  TireFR.Out/1 -> Kinetics/6
  TireFL.Out/1 -> Kinetics/5
  Demux4/1 -> Bus Creator/1  "Car Trq_T2WFL"
  Demux4/2 -> Bus Creator/2  "Car Trq_T2WFR"
  Demux4/3 -> Bus Creator/3  "Car Trq_T2WRL"
  Demux4/4 -> Bus Creator/4  "Car Trq_T2WRR"
  Bus Creator/1 -> Car.Trq_T2W/1
  Bus Creator4/1 -> WheelCarrier.Misc/1
  Demux3/4 -> Bus Creator4/4  "car Susp FR GenFrc2"
  Demux3/3 -> Bus Creator4/3  "car Susp FL GenFrc2"
  Demux3/2 -> Bus Creator4/2  "car Susp FR GenInert2"
  Demux3/1 -> Bus Creator4/1  "car Susp FL GenInert2"
  Car.Load/1 -> Kinetics/4
  Kinetics/4 -> Demux2/1
  Bus Creator3/1 -> Car.Fr1/1
  Demux2/6 -> Bus Creator3/6  "Car Fr1 rvz"
  Demux2/5 -> Bus Creator3/5  "Car Fr1 rvy"
  Demux2/4 -> Bus Creator3/4  "Car Fr1 rvx"
  Demux2/3 -> Bus Creator3/3  "Car Fr1 rz"
  Demux2/2 -> Bus Creator3/2  "Car Fr1 ry"
  Demux2/1 -> Bus Creator3/1  "Car Fr1 rx"
  Bus Creator2/1 -> Car.Hitch/1
  Kinetics/3 -> Demux1/1
  Demux1/6 -> Bus Creator2/6  "Car Hitch vz"
  Demux1/5 -> Bus Creator2/5  "Car Hitch vy"
  Demux1/4 -> Bus Creator2/4  "Car Hitch vx"
  Demux1/3 -> Bus Creator2/3  "Car Hitch tz"
  Demux1/2 -> Bus Creator2/2  "Car Hitch ty"
  Demux1/1 -> Bus Creator2/1  "Car Hitch tx"
  Demux/12 -> Bus Creator1/12  "Trailer Load_2 tz"
  Demux/11 -> Bus Creator1/11  "Trailer Load_2 ty"
  Demux/10 -> Bus Creator1/10  "Trailer Load_2 tx"
  Demux/9 -> Bus Creator1/9  "Trailer Load_2 mass"
  Demux/8 -> Bus Creator1/8  "Trailer Load_1 tz"
  Demux/7 -> Bus Creator1/7  "Trailer Load_1 ty"
  Demux/6 -> Bus Creator1/6  "Trailer Load_1 tx"
  Demux/5 -> Bus Creator1/5  "Trailer Load_1 mass"
  Kinetics/2 -> Demux/1
  Demux/4 -> Bus Creator1/4  "Trailer Load_0 tz"
  Demux/3 -> Bus Creator1/3  "Trailer Load_0 ty"
  Demux/2 -> Bus Creator1/2  "Trailer Load_0 tx"
  Demux/1 -> Bus Creator1/1  "Trailer Load_0 mass"
  Bus Creator1/1 -> Trailer.Load/1
  Car.Virtual/1 -> Kinetics/2
  Car.Aero/1 -> Kinetics/3
  Kinetics/1 -> Sync_Out/1
  Sync_In/1 -> Kinetics/1
  FBuf/1 -> Kinetics/12

== system PTMotorCU/CarMaker/IPG Vehicle/CarAndTrailer/Steering ==
  note: When replacing the entire steering system,
      | be sure to add '-disablesteering' to the command line arguments
      | in the CarMaker Model Configuration block.
  Sync_In : Inport  OutDataType=sfix(16)  OutScaling=2^0
  VhclCtrl.Steering : Inport  Port=2  OutDataType=sfix(16)  OutScaling=2^0
  Bus Creator1 : BusCreator  Inputs=16
  Bus Creator2 : BusCreator
  Demux : Demux  Outputs=20
  Steering : S-Function  FunctionName=CM_Sfun  Parameters='Steering'  EnableBusSupport=off
  Terminator : Terminator
  Sync_Out : Outport  OutDataType=sfix(16)  OutScaling=2^0
  Steer.IF : Outport  Port=2  OutDataType=sfix(16)  OutScaling=2^0
  wires:
  Demux/5 -> Bus Creator1/5  "Steering IF TrqStatic"
  Demux/4 -> Bus Creator1/4  "Steering IF Trq"
  Demux/3 -> Bus Creator1/3  "Steering IF AngAcc"
  Demux/2 -> Bus Creator1/2  "Steering IF AngVel"
  Demux/1 -> Bus Creator1/1  "Steering IF Ang"
  Sync_In/1 -> Steering/1
  Steering/1 -> Sync_Out/1
  VhclCtrl.Steering/1 -> Steering/2
  Demux/15 -> Bus Creator1/15  "Steering IF R qpp"
  Demux/14 -> Bus Creator1/14  "Steering IF R qp"
  Demux/13 -> Bus Creator1/13  "Steering IF R q"
  Demux/12 -> Bus Creator1/12  "Steering IF L iSteer2q"
  Demux/11 -> Bus Creator1/11  "Steering IF L qpp"
  Demux/10 -> Bus Creator1/10  "Steering IF L qp"
  Demux/9 -> Bus Creator1/9  "Steering IF L q"
  Demux/16 -> Bus Creator1/16  "Steering IF R iSteer2q"
  Bus Creator2/1 -> Terminator/1  "Steer IF (in)"
  Demux/19 -> Bus Creator2/3  "Steering IF R Frc"
  Demux/18 -> Bus Creator2/2  "Steering IF L Inert"
  Demux/17 -> Bus Creator2/1  "Steering IF L Frc"
  Demux/20 -> Bus Creator2/4  "Steering IF R Inert"
  Demux/6 -> Bus Creator1/6  "Steering IF AssistFrc"
  Demux/7 -> Bus Creator1/7  "Steering IF AssistTrqCol"
  Demux/8 -> Bus Creator1/8  "Steering IF AssistTrqPin"
  Steering/2 -> Demux/1
  Bus Creator1/1 -> Steer.IF/1

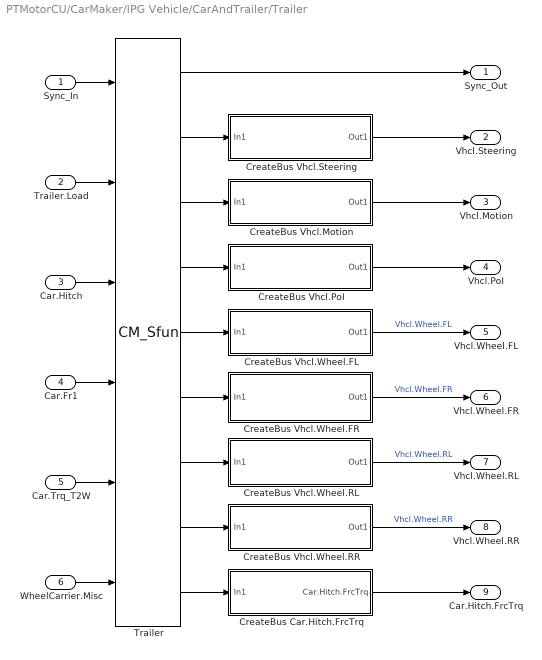
== system PTMotorCU/CarMaker/IPG Vehicle/CarAndTrailer/Trailer ==
  Sync_In : Inport  OutDataType=sfix(16)  OutScaling=2^0
  Trailer.Load : Inport  Port=2  OutDataType=sfix(16)  OutScaling=2^0
  Car.Hitch : Inport  Port=3  OutDataType=sfix(16)  OutScaling=2^0
  Car.Fr1 : Inport  Port=4  OutDataType=sfix(16)  OutScaling=2^0
  Car.Trq_T2W : Inport  Port=5  OutDataType=sfix(16)  OutScaling=2^0
  WheelCarrier.Misc : Inport  Port=6  OutDataType=sfix(16)  OutScaling=2^0
  CreateBus Car.Hitch.FrcTrq : Subsystem
  CreateBus Vhcl.Motion : Subsystem
  CreateBus Vhcl.PoI : Subsystem
  CreateBus Vhcl.Steering : Subsystem
  CreateBus Vhcl.Wheel.FL : Subsystem
  CreateBus Vhcl.Wheel.FR : Subsystem
  CreateBus Vhcl.Wheel.RL : Subsystem
  CreateBus Vhcl.Wheel.RR : Subsystem
  Trailer : S-Function  FunctionName=CM_Sfun  Parameters='Trailer'  EnableBusSupport=off
  Sync_Out : Outport  OutDataType=sfix(16)  OutScaling=2^0
  Vhcl.Steering : Outport  Port=2  OutDataType=sfix(16)  OutScaling=2^0
  Vhcl.Motion : Outport  Port=3  OutDataType=sfix(16)  OutScaling=2^0
  Vhcl.PoI : Outport  Port=4  OutDataType=sfix(16)  OutScaling=2^0
  Vhcl.Wheel.FL : Outport  Port=5  OutDataType=sfix(16)  OutScaling=2^0
  Vhcl.Wheel.FR : Outport  Port=6  OutDataType=sfix(16)  OutScaling=2^0
  Vhcl.Wheel.RL : Outport  Port=7  OutDataType=sfix(16)  OutScaling=2^0
  Vhcl.Wheel.RR : Outport  Port=8  OutDataType=sfix(16)  OutScaling=2^0
  Car.Hitch.FrcTrq : Outport  Port=9  OutDataType=sfix(16)  OutScaling=2^0
  wires:
  Sync_In/1 -> Trailer/1
  Trailer/1 -> Sync_Out/1
  Trailer.Load/1 -> Trailer/2
  Car.Hitch/1 -> Trailer/3
  Car.Fr1/1 -> Trailer/4
  CreateBus Car.Hitch.FrcTrq/1(Car.Hitch.FrcTrq) -> Car.Hitch.FrcTrq/1
  WheelCarrier.Misc/1 -> Trailer/6
  Car.Trq_T2W/1 -> Trailer/5
  CreateBus Vhcl.Motion/1(Out1) -> Vhcl.Motion/1
  CreateBus Vhcl.PoI/1(Out1) -> Vhcl.PoI/1
  CreateBus Vhcl.Wheel.FL/1(Out1) -> Vhcl.Wheel.FL/1  "Vhcl.Wheel.FL"
  CreateBus Vhcl.Wheel.FR/1(Out1) -> Vhcl.Wheel.FR/1  "Vhcl.Wheel.FR"
  CreateBus Vhcl.Wheel.RL/1(Out1) -> Vhcl.Wheel.RL/1  "Vhcl.Wheel.RL"
  CreateBus Vhcl.Wheel.RR/1(Out1) -> Vhcl.Wheel.RR/1  "Vhcl.Wheel.RR"
  Trailer/8 -> CreateBus Vhcl.Wheel.RR/1(In1)
  Trailer/9 -> CreateBus Car.Hitch.FrcTrq/1(In1)
  Trailer/7 -> CreateBus Vhcl.Wheel.RL/1(In1)
  Trailer/6 -> CreateBus Vhcl.Wheel.FR/1(In1)
  Trailer/5 -> CreateBus Vhcl.Wheel.FL/1(In1)
  Trailer/4 -> CreateBus Vhcl.PoI/1(In1)
  Trailer/3 -> CreateBus Vhcl.Motion/1(In1)
  CreateBus Vhcl.Steering/1(Out1) -> Vhcl.Steering/1
  Trailer/2 -> CreateBus Vhcl.Steering/1(In1)

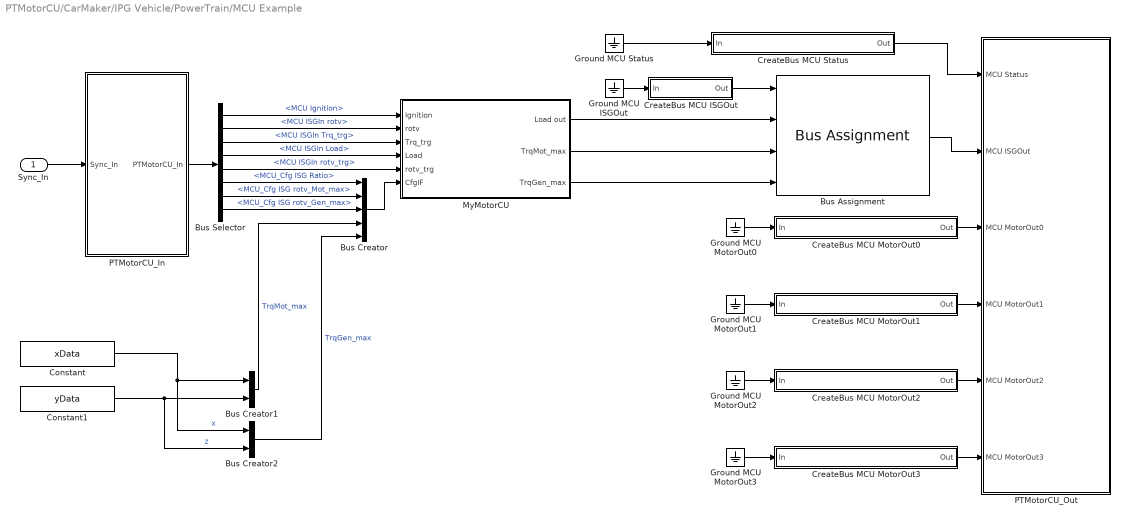
== system PTMotorCU/CarMaker/IPG Vehicle/PowerTrain/MCU Example ==
  Sync_In : Inport  OutDataType=sfix(16)  OutScaling=2^0
  Bus Assignment : BusAssignment  AssignedSignals=MCU ISGOut Load,MCU ISGOut TrqMot_max,MCU ISGOut TrqGen_max
  Bus Creator : BusCreator  Inputs=5
  Bus Creator1 : BusCreator  Inputs=2
  Bus Creator2 : BusCreator  Inputs=2
  Bus Selector : BusSelector  OutputSignals=MCU Ignition,MCU ISGIn.MCU ISGIn rotv,MCU ISGIn.MCU ISGIn Trq_trg,MCU ISGOut.MCU ISGIn Load,MCU ISGIn.MCU ISGIn rotv_trg,MCU_Cfg ISG.MCU_Cfg ISG Ratio,MCU_Cfg ISG.MCU_Cfg ISG rotv_Mot_max,MCU_Cfg ISG.MCU_Cfg ISG rotv_Gen_max
  Constant : Constant  Value=xData  OutDataType=fixdt(1, 16)  OutScaling=2^0
  Constant1 : Constant  Value=yData  OutDataType=fixdt(1, 16)  OutScaling=2^0
  CreateBus MCU ISGOut : Subsystem
  CreateBus MCU MotorOut0 : Subsystem
  CreateBus MCU MotorOut1 : Subsystem
  CreateBus MCU MotorOut2 : Subsystem
  CreateBus MCU MotorOut3 : Subsystem
  CreateBus MCU Status : Subsystem
  Ground MCU ISGOut : Ground
  Ground MCU MotorOut{0..3} (4 alike) : Ground
  Ground MCU Status : Ground
  MyMotorCU : Subsystem
  PTMotorCU_In : Subsystem
  PTMotorCU_Out : Subsystem
  wires:
  Ground MCU Status/1 -> CreateBus MCU Status/1(In)
  CreateBus MCU Status/1(Out) -> PTMotorCU_Out/1(MCU Status)
  Ground MCU MotorOut0/1 -> CreateBus MCU MotorOut0/1(In)
  CreateBus MCU MotorOut0/1(Out) -> PTMotorCU_Out/3(MCU MotorOut0)
  Ground MCU MotorOut1/1 -> CreateBus MCU MotorOut1/1(In)
  CreateBus MCU MotorOut1/1(Out) -> PTMotorCU_Out/4(MCU MotorOut1)
  Ground MCU MotorOut2/1 -> CreateBus MCU MotorOut2/1(In)
  CreateBus MCU MotorOut2/1(Out) -> PTMotorCU_Out/5(MCU MotorOut2)
  Ground MCU MotorOut3/1 -> CreateBus MCU MotorOut3/1(In)
  CreateBus MCU MotorOut3/1(Out) -> PTMotorCU_Out/6(MCU MotorOut3)
  Bus Selector/2 -> MyMotorCU/2(rotv)  "<MCU ISGIn rotv>"
  Bus Selector/3 -> MyMotorCU/3(Trq_trg)  "<MCU ISGIn Trq_trg>"
  Bus Creator/1 -> MyMotorCU/6(CfgIF)
  Bus Selector/6 -> Bus Creator/1  "<MCU_Cfg ISG Ratio>"
  Bus Creator1/1 -> Bus Creator/4  "TrqMot_max"
  Bus Selector/7 -> Bus Creator/2  "<MCU_Cfg ISG rotv_Mot_max>"
  Bus Selector/8 -> Bus Creator/3  "<MCU_Cfg ISG rotv_Gen_max>"
  Bus Selector/4 -> MyMotorCU/4(Load)  "<MCU ISGIn Load>"
  Bus Selector/5 -> MyMotorCU/5(rotv_trg)  "<MCU ISGIn rotv_trg>"
  Sync_In/1 -> PTMotorCU_In/1(Sync_In)
  PTMotorCU_In/1(PTMotorCU_In) -> Bus Selector/1
  Bus Selector/1 -> MyMotorCU/1(Ignition)  "<MCU Ignition>"
  Bus Creator2/1 -> Bus Creator/5  "TrqGen_max"
  Constant/1 -> Bus Creator1/1, Bus Creator2/1  "x"
  Constant1/1 -> Bus Creator1/2, Bus Creator2/2  "z"
  MyMotorCU/1(Load out) -> Bus Assignment/2
  MyMotorCU/2(TrqMot_max) -> Bus Assignment/3
  MyMotorCU/3(TrqGen_max) -> Bus Assignment/4
  Ground MCU ISGOut/1 -> CreateBus MCU ISGOut/1(In)
  CreateBus MCU ISGOut/1(Out) -> Bus Assignment/1
  Bus Assignment/1 -> PTMotorCU_Out/2(MCU ISGOut)

== system PTMotorCU/CarMaker/IPG Vehicle/CarAndTrailer/CarAndTrailerUpd/CreateBus Brake.IF.In ==
  In : Inport
  BusCreator : BusCreator  Inputs=9
  Demux : Demux  Outputs=9
  Out : Outport
  wires:
  In/1 -> Demux/1
  BusCreator/1 -> Out/1
  Demux/1 -> BusCreator/1  "Brake IF T_env"
  Demux/2 -> BusCreator/2  "Brake IF Trq_Reg_max FL"
  Demux/3 -> BusCreator/3  "Brake IF Trq_Reg_max FR"
  Demux/4 -> BusCreator/4  "Brake IF Trq_Reg_max RL"
  Demux/5 -> BusCreator/5  "Brake IF Trq_Reg_max RR"
  Demux/6 -> BusCreator/6  "Brake IF Trq_Reg FL"
  Demux/7 -> BusCreator/7  "Brake IF Trq_Reg FR"
  Demux/8 -> BusCreator/8  "Brake IF Trq_Reg RL"
  Demux/9 -> BusCreator/9  "Brake IF Trq_Reg RR"

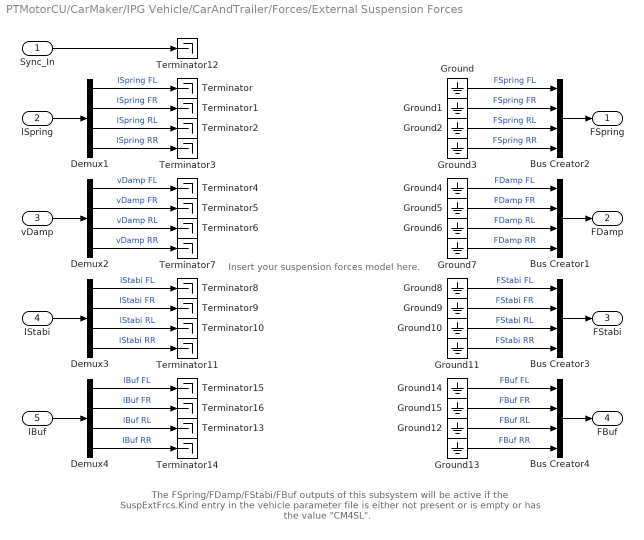
== system PTMotorCU/CarMaker/IPG Vehicle/CarAndTrailer/Forces/External Suspension Forces ==
  note: Insert your suspension forces model here.
  note: The FSpring/FDamp/FStabi/FBuf outputs of this subsystem will be
      | active if the SuspExtFrcs.Kind entry in the vehicle parameter file
      | is either not present or is empty or has the value "CM4SL".
  Sync_In : Inport  OutDataType=sfix(16)  OutScaling=2^0
  lSpring : Inport  Port=2  OutDataType=sfix(16)  OutScaling=2^0
  vDamp : Inport  Port=3  OutDataType=sfix(16)  OutScaling=2^0
  lStabi : Inport  Port=4  OutDataType=sfix(16)  OutScaling=2^0
  lBuf : Inport  Port=5  OutDataType=sfix(16)  OutScaling=2^0
  Bus Creator{1..4} (4 alike) : BusCreator
  Demux{1..4} (4 alike) : Demux
  Ground{,1..15} (16 alike) : Ground
  Terminator{,1..16} (17 alike) : Terminator
  FSpring : Outport  OutDataType=sfix(16)  OutScaling=2^0
  FDamp : Outport  Port=2  OutDataType=sfix(16)  OutScaling=2^0
  FStabi : Outport  Port=3  OutDataType=sfix(16)  OutScaling=2^0
  FBuf : Outport  Port=4  OutDataType=sfix(16)  OutScaling=2^0
  wires:
  Bus Creator3/1 -> FStabi/1
  Ground11/1 -> Bus Creator3/4  "FStabi RR"
  Ground10/1 -> Bus Creator3/3  "FStabi RL"
  Ground9/1 -> Bus Creator3/2  "FStabi FR"
  Ground8/1 -> Bus Creator3/1  "FStabi FL"
  Bus Creator1/1 -> FDamp/1
  Ground7/1 -> Bus Creator1/4  "FDamp RR"
  Ground6/1 -> Bus Creator1/3  "FDamp RL"
  Ground5/1 -> Bus Creator1/2  "FDamp FR"
  Ground4/1 -> Bus Creator1/1  "FDamp FL"
  Ground3/1 -> Bus Creator2/4  "FSpring RR"
  Ground2/1 -> Bus Creator2/3  "FSpring RL"
  Ground1/1 -> Bus Creator2/2  "FSpring FR"
  Ground/1 -> Bus Creator2/1  "FSpring FL"
  Bus Creator2/1 -> FSpring/1
  Demux2/4 -> Terminator7/1  "vDamp RR"
  Demux2/3 -> Terminator6/1  "vDamp RL"
  Demux2/2 -> Terminator5/1  "vDamp FR"
  Demux2/1 -> Terminator4/1  "vDamp FL"
  Demux1/4 -> Terminator3/1  "lSpring RR"
  Demux1/3 -> Terminator2/1  "lSpring RL"
  Demux1/2 -> Terminator1/1  "lSpring FR"
  Demux1/1 -> Terminator/1  "lSpring FL"
  Demux3/4 -> Terminator11/1  "lStabi RR"
  Demux3/3 -> Terminator10/1  "lStabi RL"
  Demux3/2 -> Terminator9/1  "lStabi FR"
  Demux3/1 -> Terminator8/1  "lStabi FL"
  lStabi/1 -> Demux3/1
  vDamp/1 -> Demux2/1
  lSpring/1 -> Demux1/1
  Sync_In/1 -> Terminator12/1
  Bus Creator4/1 -> FBuf/1
  Ground13/1 -> Bus Creator4/4  "FBuf RR"
  Ground12/1 -> Bus Creator4/3  "FBuf RL"
  Ground15/1 -> Bus Creator4/2  "FBuf FR"
  Ground14/1 -> Bus Creator4/1  "FBuf FL"
  Demux4/4 -> Terminator14/1  "lBuf RR"
  Demux4/3 -> Terminator13/1  "lBuf RL"
  Demux4/2 -> Terminator16/1  "lBuf FR"
  Demux4/1 -> Terminator15/1  "lBuf FL"
  lBuf/1 -> Demux4/1

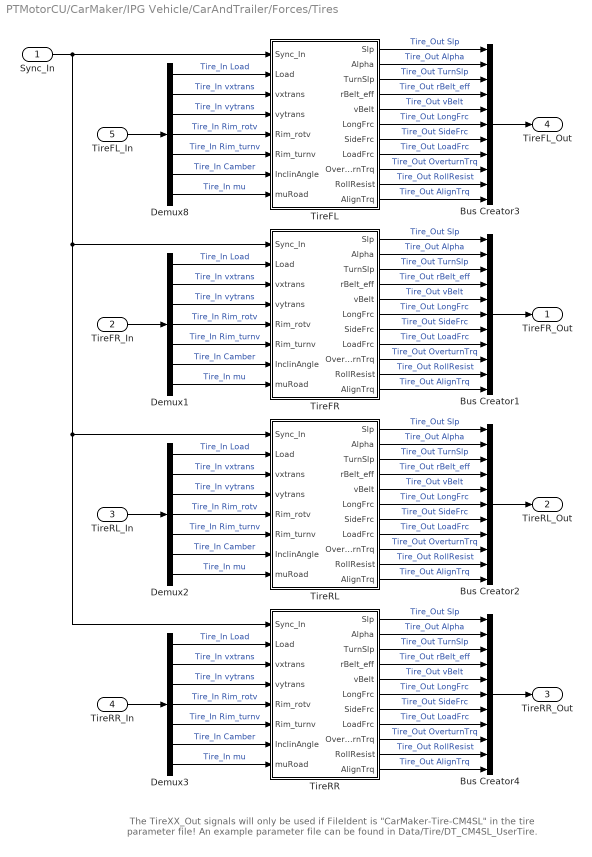
== system PTMotorCU/CarMaker/IPG Vehicle/CarAndTrailer/Forces/Tires ==
  note: The TireXX_Out signals will only be used if FileIdent is "CarMaker-Tire-CM4SL" in the tire parameter file!
      | An example parameter file can be found in Data/Tire/DT_CM4SL_UserTire.
  Sync_In : Inport  OutDataType=sfix(16)  OutScaling=2^0
  TireFR_In : Inport  Port=2  OutDataType=sfix(16)  OutScaling=2^0
  TireRL_In : Inport  Port=3  OutDataType=sfix(16)  OutScaling=2^0
  TireRR_In : Inport  Port=4  OutDataType=sfix(16)  OutScaling=2^0
  TireFL_In : Inport  Port=5  OutDataType=sfix(16)  OutScaling=2^0
  Bus Creator{1..4} (4 alike) : BusCreator  Inputs=11
  Demux{1..3,8} (4 alike) : Demux  Outputs=7
  TireFL : Subsystem
  TireFR : Subsystem
  TireRL : Subsystem
  TireRR : Subsystem
  TireFR_Out : Outport  OutDataType=sfix(16)  OutScaling=2^0
  TireRL_Out : Outport  Port=2  OutDataType=sfix(16)  OutScaling=2^0
  TireRR_Out : Outport  Port=3  OutDataType=sfix(16)  OutScaling=2^0
  TireFL_Out : Outport  Port=4  OutDataType=sfix(16)  OutScaling=2^0
  wires:
  TireRR_In/1 -> Demux3/1
  TireRL_In/1 -> Demux2/1
  TireFR_In/1 -> Demux1/1
  Bus Creator3/1 -> TireFL_Out/1
  TireFL/2(Alpha) -> Bus Creator3/2  "Tire_Out Alpha"
  TireFL/1(Slp) -> Bus Creator3/1  "Tire_Out Slp"
  TireFL/3(TurnSlp) -> Bus Creator3/3  "Tire_Out TurnSlp"
  TireFL/4(rBelt_eff) -> Bus Creator3/4  "Tire_Out rBelt_eff"
  TireFL/5(vBelt) -> Bus Creator3/5  "Tire_Out vBelt"
  TireFL/6(LongFrc) -> Bus Creator3/6  "Tire_Out LongFrc"
  TireFL/7(SideFrc) -> Bus Creator3/7  "Tire_Out SideFrc"
  TireFL/8(LoadFrc) -> Bus Creator3/8  "Tire_Out LoadFrc"
  TireFL/9(OverturnTrq) -> Bus Creator3/9  "Tire_Out OverturnTrq"
  TireFL/10(RollResist) -> Bus Creator3/10  "Tire_Out RollResist"
  TireFL/11(AlignTrq) -> Bus Creator3/11  "Tire_Out AlignTrq"
  Demux8/3 -> TireFL/4(vytrans)  "Tire_In vytrans"
  Demux8/2 -> TireFL/3(vxtrans)  "Tire_In vxtrans"
  Demux8/6 -> TireFL/7(InclinAngle)  "Tire_In Camber"
  Demux8/7 -> TireFL/8(muRoad)  "Tire_In mu"
  Demux8/1 -> TireFL/2(Load)  "Tire_In Load"
  TireFL_In/1 -> Demux8/1
  Demux8/4 -> TireFL/5(Rim_rotv)  "Tire_In Rim_rotv"
  Demux8/5 -> TireFL/6(Rim_turnv)  "Tire_In Rim_turnv"
  TireFR/2(Alpha) -> Bus Creator1/2  "Tire_Out Alpha"
  TireFR/1(Slp) -> Bus Creator1/1  "Tire_Out Slp"
  TireFR/3(TurnSlp) -> Bus Creator1/3  "Tire_Out TurnSlp"
  TireFR/4(rBelt_eff) -> Bus Creator1/4  "Tire_Out rBelt_eff"
  TireFR/5(vBelt) -> Bus Creator1/5  "Tire_Out vBelt"
  TireFR/6(LongFrc) -> Bus Creator1/6  "Tire_Out LongFrc"
  TireFR/7(SideFrc) -> Bus Creator1/7  "Tire_Out SideFrc"
  TireFR/8(LoadFrc) -> Bus Creator1/8  "Tire_Out LoadFrc"
  TireFR/9(OverturnTrq) -> Bus Creator1/9  "Tire_Out OverturnTrq"
  TireFR/10(RollResist) -> Bus Creator1/10  "Tire_Out RollResist"
  TireFR/11(AlignTrq) -> Bus Creator1/11  "Tire_Out AlignTrq"
  Demux1/3 -> TireFR/4(vytrans)  "Tire_In vytrans"
  Demux1/2 -> TireFR/3(vxtrans)  "Tire_In vxtrans"
  Demux1/6 -> TireFR/7(InclinAngle)  "Tire_In Camber"
  Demux1/7 -> TireFR/8(muRoad)  "Tire_In mu"
  Demux1/1 -> TireFR/2(Load)  "Tire_In Load"
  Demux1/4 -> TireFR/5(Rim_rotv)  "Tire_In Rim_rotv"
  Demux1/5 -> TireFR/6(Rim_turnv)  "Tire_In Rim_turnv"
  TireRL/2(Alpha) -> Bus Creator2/2  "Tire_Out Alpha"
  TireRL/1(Slp) -> Bus Creator2/1  "Tire_Out Slp"
  TireRL/3(TurnSlp) -> Bus Creator2/3  "Tire_Out TurnSlp"
  TireRL/4(rBelt_eff) -> Bus Creator2/4  "Tire_Out rBelt_eff"
  TireRL/5(vBelt) -> Bus Creator2/5  "Tire_Out vBelt"
  TireRL/6(LongFrc) -> Bus Creator2/6  "Tire_Out LongFrc"
  TireRL/7(SideFrc) -> Bus Creator2/7  "Tire_Out SideFrc"
  TireRL/8(LoadFrc) -> Bus Creator2/8  "Tire_Out LoadFrc"
  TireRL/9(OverturnTrq) -> Bus Creator2/9  "Tire_Out OverturnTrq"
  TireRL/10(RollResist) -> Bus Creator2/10  "Tire_Out RollResist"
  TireRL/11(AlignTrq) -> Bus Creator2/11  "Tire_Out AlignTrq"
  Demux2/3 -> TireRL/4(vytrans)  "Tire_In vytrans"
  Demux2/2 -> TireRL/3(vxtrans)  "Tire_In vxtrans"
  Demux2/6 -> TireRL/7(InclinAngle)  "Tire_In Camber"
  Demux2/7 -> TireRL/8(muRoad)  "Tire_In mu"
  Demux2/1 -> TireRL/2(Load)  "Tire_In Load"
  Demux2/4 -> TireRL/5(Rim_rotv)  "Tire_In Rim_rotv"
  Demux2/5 -> TireRL/6(Rim_turnv)  "Tire_In Rim_turnv"
  TireRR/2(Alpha) -> Bus Creator4/2  "Tire_Out Alpha"
  TireRR/1(Slp) -> Bus Creator4/1  "Tire_Out Slp"
  TireRR/3(TurnSlp) -> Bus Creator4/3  "Tire_Out TurnSlp"
  TireRR/4(rBelt_eff) -> Bus Creator4/4  "Tire_Out rBelt_eff"
  TireRR/5(vBelt) -> Bus Creator4/5  "Tire_Out vBelt"
  TireRR/6(LongFrc) -> Bus Creator4/6  "Tire_Out LongFrc"
  TireRR/7(SideFrc) -> Bus Creator4/7  "Tire_Out SideFrc"
  TireRR/8(LoadFrc) -> Bus Creator4/8  "Tire_Out LoadFrc"
  TireRR/9(OverturnTrq) -> Bus Creator4/9  "Tire_Out OverturnTrq"
  TireRR/10(RollResist) -> Bus Creator4/10  "Tire_Out RollResist"
  TireRR/11(AlignTrq) -> Bus Creator4/11  "Tire_Out AlignTrq"
  Demux3/3 -> TireRR/4(vytrans)  "Tire_In vytrans"
  Demux3/2 -> TireRR/3(vxtrans)  "Tire_In vxtrans"
  Demux3/6 -> TireRR/7(InclinAngle)  "Tire_In Camber"
  Demux3/7 -> TireRR/8(muRoad)  "Tire_In mu"
  Demux3/1 -> TireRR/2(Load)  "Tire_In Load"
  Demux3/4 -> TireRR/5(Rim_rotv)  "Tire_In Rim_rotv"
  Demux3/5 -> TireRR/6(Rim_turnv)  "Tire_In Rim_turnv"
  Bus Creator1/1 -> TireFR_Out/1
  Bus Creator2/1 -> TireRL_Out/1
  Bus Creator4/1 -> TireRR_Out/1
  Sync_In/1 -> TireFL/1(Sync_In), TireFR/1(Sync_In), TireRL/1(Sync_In), TireRR/1(Sync_In)
